simulink model "problem4"  (R2020b)
settings: Solver=VariableStepAuto  StartTime=0.0  StopTime=10.0  RelTol=1e-3
settings Model: Creator=ARPITA  LastModifiedBy=ARPITA

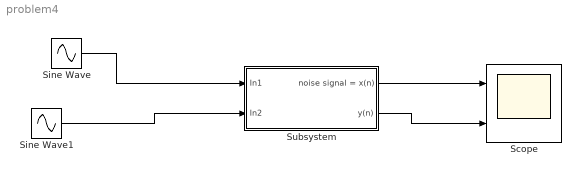
== system problem4 ==
  Scope : Scope  NumInputPorts=2
  Sine Wave : Sin  SampleTime=0
  Sine Wave1 : Sin  Amplitude=0.05  Frequency=100  SampleTime=0
  Subsystem : Subsystem
  wires:
  Sine Wave/1 -> Subsystem/1(In1)
  Sine Wave1/1 -> Subsystem/2(In2)
  Subsystem/1(noise signal = x(n)) -> Scope/1
  Subsystem/2(y(n)) -> Scope/2

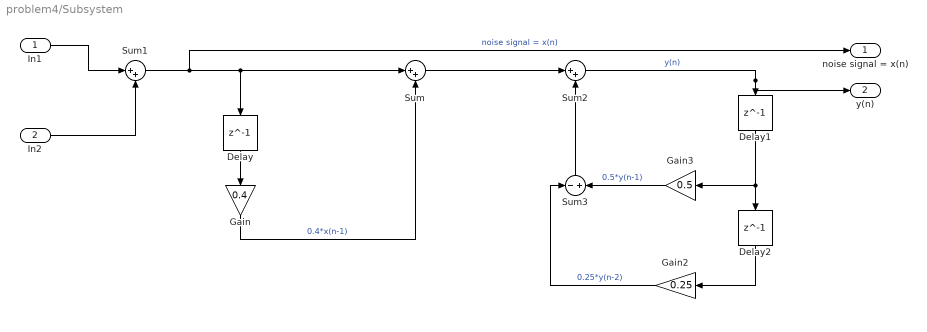
== system problem4/Subsystem ==
  In1 : Inport
  In2 : Inport  Port=2
  Delay : Delay  DelayLength=1  InitialCondition=0
  Delay1 : Delay  DelayLength=1  InitialCondition=0
  Delay2 : Delay  DelayLength=1  InitialCondition=0
  Gain : Gain  Gain=0.4
  Gain2 : Gain  Gain=0.25
  Gain3 : Gain  Gain=0.5
  Sum : Sum  Inputs=|++
  Sum1 : Sum  Inputs=|++
  Sum2 : Sum  Inputs=|++
  Sum3 : Sum  Inputs=-+
  noise signal = x(n) : Outport
  y(n) : Outport  Port=2
  wires:
  Delay2/1 -> Gain2/1
  Gain2/1 -> Sum3/1  "0.25*y(n-2)"
  Gain/1 -> Sum/2  "0.4*x(n-1)"
  Delay1/1 -> Gain3/1, Delay2/1
  Delay/1 -> Gain/1
  Sum/1 -> Sum2/1
  Sum2/1 -> y(n)/1, Delay1/1  "y(n)"
  Gain3/1 -> Sum3/2  "0.5*y(n-1)"
  Sum3/1 -> Sum2/2
  Sum1/1 -> noise signal = x(n)/1, Sum/1, Delay/1  "noise signal = x(n)"
  In2/1 -> Sum1/2
  In1/1 -> Sum1/1
